simulink model "D_20231120_Modell_Inbetriebnahme_BreakOutBox_Jetson"  (R2022b)
settings: Solver=ode1  StartTime=0.0  StopTime=inf  FixedStep=Ts  RelTol=1e-3
PreLoadFcn:
  | pulsePeriod = 0.05;
  | 
  | Ts = 0.001;
  | 
  | FPGA_Frequency = 75000000;
  | 
  | ts_IO691 = 5e-3;
PostLoadFcn:
  | ewolfSetUp
InitFcn:
  | pulsePeriod = 0.05;
  | 
  | Ts = 0.001;
  | 
  | FPGA_Frequency = 75000000;
  | 
  | ts_IO691 = 5e-3;
StopFcn:
  | Simulink.sdi.clearPreferences;
  | if isfile(['sdi_view_',bdroot,'.mldatx'])
  | Simulink.sdi.view;
  | pause(3);
  | Simulink.sdi.loadView(['sdi_view_',bdroot,]);
  | end
model workspace (MAT data in the model file):
  MaxDreh = 1
values from neighbouring files (symbols this model uses):
  max_ac = 2    [ewolfSetUp.m]
  min_ac = -3    [ewolfSetUp.m]
  PredictionHorizon = 30    [ewolfSetUp.m]
undefined symbols (not defined in the file or in its folder): canChannel, DiscIntNeverNeededParam, Ended, HS, IO291, IO397, max_steer_car, min_steer_car, sigbuilder_block, Single
libraries: lllalib x255, canmsglib x146, simulink x42, speedgoatlib_IO191 x5, speedgoatlib_IO291 x5, slrealtimeiplib x3, speedgoatlib_IO691 x3, slrealtimeutilitieslib x2, spsEdgeDetectorLib x1, simulink_extras x1, speedgoatlib_fpga_dio x1, speedgoatlib_fpga_quadrature x1
(part 7 of 8)

== system D_20231120_Modell_Inbetriebnahme_BreakOutBox_Jetson/Lenkung Steuerung/Beobachter und Begrenzer/Lenkwingelgeschwindigkeitsbegrenzer ==
  "Drehmomvor. norm. " : Inport
  LenkDrehmomentMaxNomiert : Inport  Port=2
  Constant : Constant  Value=0
  Saturation : Saturate  UpperLimit=1  LowerLimit=0
  Saturation Dynamic : simulink/Discontinuities/Saturation Dynamic  OutMin=[]  OutMax=[]  OutDataTypeStr=Inherit: Same as second input  OutDataType=fixdt(1, 16)  OutScaling=2^-10  DoSatur=off
  Saturation1 : Saturate  UpperLimit=1  LowerLimit=0
  Terminator : Terminator
  Drehmoment norm. begr. : Outport
  wires:
  Saturation1/1 -> Drehmoment norm. begr./1
  "Drehmomvor. norm. "/1 -> Saturation Dynamic/2, Saturation1/1
  Constant/1 -> Saturation Dynamic/3
  LenkDrehmomentMaxNomiert/1 -> Saturation/1
  Saturation/1 -> Saturation Dynamic/1
  Saturation Dynamic/1 -> Terminator/1  "Drehmoment norm. begr. Test"

== system D_20231120_Modell_Inbetriebnahme_BreakOutBox_Jetson/Lenkung Steuerung/Beobachter und Begrenzer/Lenkwinkelbegrenzer ==
  Lenkwinkel nomiert : Inport
  Drehmomvor. norm. : Inport  Port=2
  "Maximaler Lenkwinkel normiert und Geschwindigkeitsabhängig " : Inport  Port=3
  Constant : Constant
  Constant1 : Constant  Value=0.5
  IC1 : InitialCondition  Value=0.5
  Lamp : LampBlock  LabelPosition=Hide
  Lamp1 : LampBlock  LabelPosition=Hide
  Lamp2 : LampBlock  LabelPosition=Hide
  RT : RateTransition  OutPortSampleTime=0.001
  Relational Operator : RelationalOperator  OutDataTypeStr=boolean  RndMeth=Simplest  InputSameDT=off
  Relational Operator1 : RelationalOperator  Operator=<=  OutDataTypeStr=boolean  RndMeth=Simplest  InputSameDT=off
  Split pos. and neg. Drehmoment : Subsystem
  Sum : Sum  Inputs=|+-
  Switch : Switch  Criteria=u2 > Threshold  SaturateOnIntegerOverflow=off  InputSameDT=off
  Switch1 : Switch  Criteria=u2 > Threshold  SaturateOnIntegerOverflow=off  InputSameDT=off
  Switch2 : Switch  Criteria=u2 > Threshold  SaturateOnIntegerOverflow=off  InputSameDT=off
  "Drehmomvor. norm. " : Outport
  wires:
  Drehmomvor. norm./1 -> Split pos. and neg. Drehmoment/1(Drehmomvor. norm.)
  Switch/1 -> Switch2/3
  Switch1/1 -> Switch2/1
  Split pos. and neg. Drehmoment/2(bool Welle) -> Switch2/2
  Split pos. and neg. Drehmoment/3(neg. Welle) -> Switch/1
  Relational Operator/1 -> Switch/2
  Relational Operator1/1 -> RT/1
  Lenkwinkel nomiert/1 -> Relational Operator/1, Relational Operator1/1
  "Maximaler Lenkwinkel normiert und Geschwindigkeitsabhängig "/1 -> Sum/2, Relational Operator1/2
  Constant1/1 -> Switch1/3, Switch/3
  RT/1 -> Switch1/2
  Split pos. and neg. Drehmoment/1(pos. Welle) -> Switch1/1
  Sum/1 -> Relational Operator/2
  Constant/1 -> Sum/1
  IC1/1 -> "Drehmomvor. norm. "/1
  Switch2/1 -> IC1/1

== system D_20231120_Modell_Inbetriebnahme_BreakOutBox_Jetson/Lenkung Steuerung/Beobachter und Begrenzer/Subsystem1 ==
  Geschwindigkeit : Inport
  Lenkwinkel : Inport  Port=2
  Constant : Constant  Value=10
  Derivative : Derivative
  MATLAB Function : MATLAB Function  TreatAsAtomicUnit=on
  MATLAB Function1 : MATLAB Function  TreatAsAtomicUnit=on
  Product : Product
  lenkradwinkelMaxNomiert : Outport
  LenkDrehmomentMaxNomiert : Outport  Port=2
  wires:
  MATLAB Function1/1(LenkDrehmomentMaxNomiert) -> LenkDrehmomentMaxNomiert/1  "LenkDrehmomentMaxNomiert"
  MATLAB Function/1(lenkradwinkelMaxNomiert) -> lenkradwinkelMaxNomiert/1  "lenkradwinkelMaxNomiert"
  Lenkwinkel/1 -> MATLAB Function/1(Lenkwinkel), Derivative/1
  Derivative/1 -> MATLAB Function1/1(Lenkwinkelgeschwindigkeit)  "LenkradwinkelGeschwindigkeit"
  Geschwindigkeit/1 -> Product/1
  Product/1 -> MATLAB Function/2(Fahrzeuggeschwindigkeit), MATLAB Function1/2(Fahrzeuggeschwindigkeit)
  Constant/1 -> Product/2

== system D_20231120_Modell_Inbetriebnahme_BreakOutBox_Jetson/Lenkung Steuerung/Lenkmomentsimulationssignalgeber/Signal Builder ==
  Demux : Demux  Tag=STV Demux  Outputs=5
      settings: DisplayOption=none
  FromWs : FromWorkspace  Tag=STV FromWs  VariableName=tuvar
      SigBuilderData=|
      | common.afterFinalStr = 'Extrapolate'
      | common.sampleTime = 0
      | dataSet.timeRange = [0 100]
      | dataSet.name = 'Group 1'
      | sbobj.Groups.Name = 'Group 1'
      | sbobj.Groups.Signals(1).Name = 'Signal 1'
      | sbobj.Groups.Signals(1).XData = [0 5 5 10 10 15 15 20 20 25 25 30 30 35 35 40 40 45 45 50 50 55 55 60 60 65 65 70 70 75 75 80 80 85 85 90 90 95 95 100]
      | sbobj.Groups.Signals(1).YData = [0 0 0.5 0.5 0 0 -0.5 -0.5 0 0 1 1 0 0 -1 -1 0 0 1.5 1.5 0 0 -1.5 -1.5 0 0 2 2 0 0 -2 -2 -0.05 -0.05 0.25 0.25 0 0 -0.25 -0.25]
      | sbobj.Groups.Signals(2).Name = 'Signal 2'
      | sbobj.Groups.Signals(2).XData = [0 10 10 30 30 100]
      | sbobj.Groups.Signals(2).YData = [0.5 0.5 0.3 0.3 0.7 0.7]
      | sbobj.Groups.Signals(3).Name = 'Signal 3'
      | sbobj.Groups.Signals(3).XData = [0 20 40 40 60 100]
      | sbobj.Groups.Signals(3).YData = [0.5 0.5 1 0.5 0 0.5]
      | sbobj.Groups.Signals(4).Name = 'Signal 4'
      | sbobj.Groups.Signals(4).XData = [0 10 10 100]
      | sbobj.Groups.Signals(4).YData = [0 0 0.5 0.5]
      | sbobj.Groups.Signals(5).Name = 'Signal 5'
      | sbobj.Groups.Signals(5).XData = [0 20 100]
      | sbobj.Groups.Signals(5).YData = [-4 -4 4]
      | sbobj.Groups.TimeRange = [0 100]
  Signal 1 : Outport  Tag=STV Outport
  Signal 2 : Outport  Tag=STV Outport  Port=2
  Signal 3 : Outport  Tag=STV Outport  Port=3
  Signal 4 : Outport  Tag=STV Outport  Port=4
  Signal 5 : Outport  Tag=STV Outport  Port=5
  wires:
  Demux/1 -> Signal 1/1
  FromWs/1 -> Demux/1
  Demux/2 -> Signal 2/1
  Demux/3 -> Signal 3/1
  Demux/4 -> Signal 4/1
  Demux/5 -> Signal 5/1

== system D_20231120_Modell_Inbetriebnahme_BreakOutBox_Jetson/Nvidia_Jetson/LaneFollowingAndControl/Estimate Lane Center1 ==
  note: Estimate Lane Center
  Lane Detections : Inport
  Longitudinal Velocity : Inport  Port=2
  Center from Left and Right1 : Subsystem  TreatAsAtomicUnit=on
  Center from Left1 : Subsystem  TreatAsAtomicUnit=on
  Center from None1 : Subsystem  TreatAsAtomicUnit=on
  Center from Right1 : Subsystem  TreatAsAtomicUnit=on
  Delay1 : Delay  DelayLength=1
  Lane Detections5 : InportShadow
  Lane Detections6 : InportShadow
  Lane Detections7 : InportShadow
  MATLAB Function1 : MATLAB Function  TreatAsAtomicUnit=on
  Merge1 : Merge  Inputs=4
  Preview Curvature : Subsystem  VariantControl=v2
      settings: RTWFileNameOpts=Use function name
  Previewed Curvature : Outport  VectorParamsAs1DForOutWhenUnconnected=off
  Lateral Offset : Outport  Port=2  VectorParamsAs1DForOutWhenUnconnected=off
  Heading Angle : Outport  Port=3  VectorParamsAs1DForOutWhenUnconnected=off
  wires:
  Preview Curvature/1(Previewed Curvature) -> Previewed Curvature/1
  Merge1/1 -> Preview Curvature/1(Lane Center), Delay1/1
  Center from Left1/1(Center) -> Merge1/2
  Lane Detections5/1 -> Center from Left and Right1/1(Lanes)
  Center from Left and Right1/1(Center) -> Merge1/1
  Lane Detections6/1 -> Center from Left1/1(Lanes)
  Delay1/1 -> Center from None1/1(In1)
  Lane Detections/1 -> MATLAB Function1/1(lanes)
  Lane Detections7/1 -> Center from Right1/1(Lanes)
  Center from None1/1(Out1) -> Merge1/4
  Center from Right1/1(Center) -> Merge1/3
  Longitudinal Velocity/1 -> Preview Curvature/2(Longitudinal Velocity)
  Preview Curvature/3(Relative Yaw Angle) -> Heading Angle/1  "relative_yaw_angle"
  Preview Curvature/2(Lateral Deviation) -> Lateral Offset/1  "lateral_deviation"
  MATLAB Function1/1(fcnLeftAndRight()) -> Center from Left and Right1/Trigger
  MATLAB Function1/2(fcnLeftOnly()) -> Center from Left1/Trigger
  MATLAB Function1/3(fcnRightOnly()) -> Center from Right1/Trigger
  MATLAB Function1/4(fcnNone()) -> Center from None1/Trigger

== system D_20231120_Modell_Inbetriebnahme_BreakOutBox_Jetson/Nvidia_Jetson/LaneFollowingAndControl/MPC Controller ==
  Set velocity : Inport
  Longitudinal velocity : Inport  Port=2
  Curvature : Inport  Port=3
  Lateral deviation : Inport  Port=4
  Relative yaw angle : Inport  Port=5
  Initial Velocity : Constant  Value=0.1
  Path Following Control System : mpcadaslib/Path Following Control System  VariantControl=Variant2  ModelType=Use vehicle parameters  VehicleMass=m  VehicleYawInertia=Iz  LengthToFront=lf  LengthToRear=lr  FrontTireStiffness=Cf  RearTireStiffness=Cr  AccelTimeConstant=tau  EgoModelMatrixA=[-2,zeros(1,3);1,zeros(1,3);zeros(1,2),-4.4021,-12.4603;zeros(1,2),1.3913,-5.1868]  EgoModelMatrixB=[2,zeros(1,3);zeros(1,2),24.1270,15.8609]'  EgoModelMatrixC=[zeros(3,1),eye(3)]  InitialLongVel=v0_ego  TransportLag=0.1  spaceCtrl=off  DefaultSpacing=default_spacing  MinSteering=min_steer  umin_ext=off  MaxSteering=max_steer  umax_ext=off  MinAcceleration=min_ac  amin_ext=off  MaxAcceleration=max_ac  amax_ext=off  Ts=0.1  PredictionHorizon=PredictionHorizon  ControlHorizon=2  LongWeight=0.1  LateralWeight=1  AccelRateWeight=0.1  SteerRateWeight=0.1  suboptimal=off  maxiter=10  datatypeopt=double  optmode=off  trackmode=off
  Switch : Switch  Criteria=u2 > Threshold  Threshold=0.1  SaturateOnIntegerOverflow=off  InputSameDT=off
  Steering Angle : Outport  VectorParamsAs1DForOutWhenUnconnected=off
  Acceleration : Outport  Port=2  VectorParamsAs1DForOutWhenUnconnected=off
  wires:
  Lateral deviation/1 -> Path Following Control System/4
  Curvature/1 -> Path Following Control System/3
  Set velocity/1 -> Path Following Control System/1
  Path Following Control System/2 -> Steering Angle/1
  Path Following Control System/1 -> Acceleration/1
  Relative yaw angle/1 -> Path Following Control System/5
  Initial Velocity/1 -> Switch/3
  Longitudinal velocity/1 -> Switch/2, Switch/1  "Longitudinal_Velocity"
  Switch/1 -> Path Following Control System/2

== system D_20231120_Modell_Inbetriebnahme_BreakOutBox_Jetson/Freigabe/Freigabe/Detektion Fahrpedal/Moving Average ==
  In : Inport
  Divide : Product  Inputs=*/
  Sum of Elements : Sum  Inputs=+
  Tapped Delay : simulink/Discrete/Tapped Delay  vinit=0.0  samptime=-1  NumDelays=4  DelayOrder=Oldest  includeCurrent=off
  Vector Concatenate : Concatenate
  Width : Width
  Out : Outport
  wires:
  In/1 -> Vector Concatenate/1, Tapped Delay/1
  Sum of Elements/1 -> Divide/1
  Width/1 -> Divide/2
  Vector Concatenate/1 -> Sum of Elements/1, Width/1
  Divide/1 -> Out/1
  Tapped Delay/1 -> Vector Concatenate/2

== system D_20231120_Modell_Inbetriebnahme_BreakOutBox_Jetson/Freigabe/Freigabe/Detektion Fahrpedal/Moving Average1 ==
  In : Inport
  Divide : Product  Inputs=*/
  Sum of Elements : Sum  Inputs=+
  Tapped Delay : simulink/Discrete/Tapped Delay  vinit=0.0  samptime=-1  NumDelays=4  DelayOrder=Oldest  includeCurrent=off
  Vector Concatenate : Concatenate
  Width : Width
  Out : Outport
  wires:
  In/1 -> Vector Concatenate/1, Tapped Delay/1
  Sum of Elements/1 -> Divide/1
  Width/1 -> Divide/2
  Vector Concatenate/1 -> Sum of Elements/1, Width/1
  Divide/1 -> Out/1
  Tapped Delay/1 -> Vector Concatenate/2

== system D_20231120_Modell_Inbetriebnahme_BreakOutBox_Jetson/IO691/CAN Read Loop - Port 3/Enabled Subsystem/extract radar data from CAN msg stream ==
  msg : Inport
  CAN Log : canlib/CAN Log  Commented=on  BlockHandle=781.0001  FullPathFileName=loGG.mat  FileName=loGG.mat  VariableName=saveMSG  MaxNumMessages=1000  LogFrom=CAN Bus  DeviceMenu=Select a device  Device=Vector CANcaseXL 1 (Channel 1)  ObjConstructor=canChannel('Vector', 'CANcaseXL 1', 1)  SampleTime=inf
  Mux : Mux  Inputs=6
  Subsystem1 : Subsystem
  Subsystem100 : Subsystem
  extract point from CAN msg : Subsystem
  save 55 : Subsystem
  enable outP : Outport
  data : Outport  Port=2  OutDataTypeStr=double
  Radar_Punkt : Outport  Port=3
  Radar_Mode : Outport  Port=4
  wires:
  extract point from CAN msg/6(numobj) -> Mux/3
  extract point from CAN msg/4(cycle) -> Mux/2
  extract point from CAN msg/3(data) -> Radar_Punkt/1, Subsystem100/2(data)
  extract point from CAN msg/2(timestamp) -> Mux/1
  msg/1 -> extract point from CAN msg/1(msg)
  extract point from CAN msg/1(enable) -> Subsystem100/1(reset), Subsystem1/1(reset), save 55/1(reset), enable outP/1
  extract point from CAN msg/5(mode) -> Subsystem100/3(saveBool), Subsystem1/3(saveBool), save 55/3(saveBool), Radar_Mode/1
  Mux/1 -> data/1
  Subsystem100/1(Out1) -> Mux/4
  save 55/1(Out1) -> Mux/6
  Subsystem1/1(Out1) -> Mux/5
  Subsystem1/2(nextSave) -> save 55/2(data)
  Subsystem100/2(nextSave) -> Subsystem1/2(data)

== system D_20231120_Modell_Inbetriebnahme_BreakOutBox_Jetson/Lenkung Steuerung/Beobachter und Begrenzer/Lenkwinkelbegrenzer/Split pos. and neg. Drehmoment ==
  Drehmomvor. norm. : Inport
  Constant : Constant  Value=0.5
  Enabled Subsystem : Subsystem  TreatAsAtomicUnit=on
  Enabled Subsystem1 : Subsystem  TreatAsAtomicUnit=on
  Logical Operator : Logic  Operator=NOT  AllPortsSameDT=off  OutDataTypeStr=boolean
  Relational Operator : RelationalOperator  Operator=>  OutDataTypeStr=boolean  RndMeth=Simplest  InputSameDT=off
  pos. Welle : Outport
  bool Welle : Outport  Port=2
  neg. Welle : Outport  Port=3
  wires:
  Relational Operator/1 -> bool Welle/1, Logical Operator/1, Enabled Subsystem1/Enable
  Drehmomvor. norm./1 -> Enabled Subsystem/1(Drehmomentsvorgabe normiert), Relational Operator/1, Enabled Subsystem1/1(Drehmomentsvorgabe normiert)
  Constant/1 -> Relational Operator/2
  Logical Operator/1 -> Enabled Subsystem/Enable
  Enabled Subsystem1/1(Out1) -> pos. Welle/1
  Enabled Subsystem/1(Out1) -> neg. Welle/1

== system D_20231120_Modell_Inbetriebnahme_BreakOutBox_Jetson/Nvidia_Jetson/LaneFollowingAndControl/Estimate Lane Center1/Center from Left and Right1 ==
  note: Center from Left and Right
  In Bus Element : Inport  PortName=Lanes  Element=Left.Curvature
  In Bus Element2 : Inport  PortName=Lanes  Element=Left.CurvatureDerivative
  In Bus Element4 : Inport  PortName=Lanes  Element=Left.HeadingAngle
  In Bus Element6 : Inport  PortName=Lanes  Element=Left.LateralOffset
  In Bus Element1 : Inport  PortName=Lanes  Element=Right.Curvature
  In Bus Element3 : Inport  PortName=Lanes  Element=Right.CurvatureDerivative
  In Bus Element5 : Inport  PortName=Lanes  Element=Right.HeadingAngle
  In Bus Element7 : Inport  PortName=Lanes  Element=Right.LateralOffset
  function : TriggerPort  TriggerType=function-call  VariantControl=Variant
  Add{,1..3} (4 alike) : Sum
  Bus Creator : BusCreator  Inputs=4
  Gain{,1..3} (4 alike) : Gain  Gain=0.5
  Center : Outport  VectorParamsAs1DForOutWhenUnconnected=off
  wires:
  In Bus Element6/1 -> Add3/1
  In Bus Element7/1 -> Add3/2
  In Bus Element5/1 -> Add2/2
  In Bus Element4/1 -> Add2/1
  In Bus Element3/1 -> Add1/2
  In Bus Element2/1 -> Add1/1
  In Bus Element1/1 -> Add/2
  In Bus Element/1 -> Add/1
  Bus Creator/1 -> Center/1
  Gain3/1 -> Bus Creator/4  "LateralOffset"
  Add3/1 -> Gain3/1
  Gain2/1 -> Bus Creator/3  "HeadingAngle"
  Add2/1 -> Gain2/1
  Gain1/1 -> Bus Creator/2  "CurvatureDerivative"
  Add1/1 -> Gain1/1
  Gain/1 -> Bus Creator/1  "Curvature"
  Add/1 -> Gain/1

== system D_20231120_Modell_Inbetriebnahme_BreakOutBox_Jetson/Nvidia_Jetson/LaneFollowingAndControl/Estimate Lane Center1/Center from Left1 ==
  note: Curvature Derivative
      | = D[ 1 / ( 1 / (left curvature) – guard)]
      | = left curvature derivative / (1 – (left curvature) * guard)^2.
  note: Center from Left
  note: Curvature
      | = 1 / ( 1 / (left curvature) – guard)
      | = left curvature / (1 – (left curvature) * guard).
  In Bus Element : Inport  PortName=Lanes  Element=Left.Curvature
  In Bus Element2 : Inport  PortName=Lanes  Element=Left.CurvatureDerivative
  In Bus Element4 : Inport  PortName=Lanes  Element=Left.HeadingAngle
  In Bus Element6 : Inport  PortName=Lanes  Element=Left.LateralOffset
  function : TriggerPort  TriggerType=function-call  VariantControl=Variant
  Bus Creator : BusCreator  Inputs=4
  Constant : Constant  OutDataTypeStr=Inherit: Inherit via back propagation
  Divide : Product  Inputs=*/
  Divide1 : Product  Inputs=*/
  Half Lane Width Estimate : Constant  Value=1.8  OutDataTypeStr=Inherit: Inherit via back propagation
  Half Lane Width Estimate1 : Constant  Value=1.8  OutDataTypeStr=Inherit: Inherit via back propagation
  Product : Product
  Product1 : Product
  Subtract : Sum  Inputs=+-
  Subtract1 : Sum  Inputs=+-
  Center : Outport  VectorParamsAs1DForOutWhenUnconnected=off
  wires:
  Product/1 -> Subtract/2
  Half Lane Width Estimate1/1 -> Subtract1/2
  In Bus Element6/1 -> Subtract1/1  "LateralOffset"
  Product1/1 -> Divide1/2
  In Bus Element2/1 -> Divide1/1  "CurvatureDerivative"
  Constant/1 -> Subtract/1
  Half Lane Width Estimate/1 -> Product/2
  Subtract/1 -> Divide/2, Product1/1, Product1/2
  In Bus Element/1 -> Divide/1, Product/1  "Curvature"
  Subtract1/1 -> Bus Creator/4  "LateralOffset"
  In Bus Element4/1 -> Bus Creator/3  "HeadingAngle"
  Divide/1 -> Bus Creator/1  "Curvature"
  Divide1/1 -> Bus Creator/2  "CurvatureDerivative"
  Bus Creator/1 -> Center/1

== system D_20231120_Modell_Inbetriebnahme_BreakOutBox_Jetson/Nvidia_Jetson/LaneFollowingAndControl/Estimate Lane Center1/Center from None1 ==
  In1 : Inport
  function : TriggerPort  TriggerType=function-call  VariantControl=Variant
  Out1 : Outport  VectorParamsAs1DForOutWhenUnconnected=off
  wires:
  In1/1 -> Out1/1

== system D_20231120_Modell_Inbetriebnahme_BreakOutBox_Jetson/Nvidia_Jetson/LaneFollowingAndControl/Estimate Lane Center1/Center from Right1 ==
  note: Curvature Derivative
      | = D[ 1 / ( 1 / (right curvature) + guard)]
      | = right curvature derivative / (1 + (right curvature) * guard)^2
  note: Curvature
      | = 1 / ( 1 / (right curvature) + guard)
      | = right curvature / (1 + (right curvature) * guard)
  note: Center from Right
  In Bus Element : Inport  PortName=Lanes  Element=Right.Curvature
  In Bus Element2 : Inport  PortName=Lanes  Element=Right.CurvatureDerivative
  In Bus Element4 : Inport  PortName=Lanes  Element=Right.HeadingAngle
  In Bus Element6 : Inport  PortName=Lanes  Element=Right.LateralOffset
  function : TriggerPort  TriggerType=function-call  VariantControl=Variant
  Bus Creator : BusCreator  Inputs=4
  Constant : Constant  OutDataTypeStr=Inherit: Inherit via back propagation
  Divide : Product  Inputs=*/
  Divide1 : Product  Inputs=*/
  Half Lane Width Estimate : Constant  Value=1.8  OutDataTypeStr=Inherit: Inherit via back propagation
  Half Lane Width Estimate1 : Constant  Value=1.8  OutDataTypeStr=Inherit: Inherit via back propagation
  Product : Product
  Product1 : Product
  Subtract : Sum
  Subtract1 : Sum
  Center : Outport  VectorParamsAs1DForOutWhenUnconnected=off
  wires:
  Half Lane Width Estimate/1 -> Product/2
  Product/1 -> Subtract/2
  Constant/1 -> Subtract/1
  Subtract/1 -> Divide/2, Product1/1, Product1/2
  In Bus Element/1 -> Divide/1, Product/1  "Curvature"
  Bus Creator/1 -> Center/1
  Subtract1/1 -> Bus Creator/4  "LateralOffset"
  Divide/1 -> Bus Creator/1  "Curvature"
  In Bus Element6/1 -> Subtract1/1  "LateralOffset"
  Half Lane Width Estimate1/1 -> Subtract1/2
  In Bus Element4/1 -> Bus Creator/3  "HeadingAngle"
  Product1/1 -> Divide1/2
  Divide1/1 -> Bus Creator/2  "CurvatureDerivative"
  In Bus Element2/1 -> Divide1/1  "CurvatureDerivative"

== system D_20231120_Modell_Inbetriebnahme_BreakOutBox_Jetson/Nvidia_Jetson/LaneFollowingAndControl/Estimate Lane Center1/Preview Curvature ==
  Lane Center : Inport
  Longitudinal Velocity : Inport  Port=2
  Bus Selector : BusSelector  OutputSignals=Curvature,CurvatureDerivative,HeadingAngle,LateralOffset
  Data Type Conversion{,1..3} (4 alike) : DataTypeConversion  SaturateOnIntegerOverflow=off  RndMeth=Floor
  Gain : Gain  Gain=[0:0.1:PredictionHorizon*0.1]'
      settings: AttributesFormatString=|
      | ----------------------------------------
      | Gain = %<Gain>
  ISO 8855 to SAE J670E : Subsystem
  Product : Product
  Saturation : Saturate
      settings: AttributesFormatString=|
      | -------------------------------
      | UpperLimit = %<UpperLimit>
      | LowerLimit = %<LowerLimit>
  Saturation1 : Saturate  UpperLimit=0.6  LowerLimit=-0.6
      settings: AttributesFormatString=|
      | -------------------------------
      | UpperLimit = %<UpperLimit>
      | LowerLimit = %<LowerLimit>
  Saturation2 : Saturate  UpperLimit=0.15  LowerLimit=-0.15
      settings: AttributesFormatString=|
      | -------------------------------
      | UpperLimit = %<UpperLimit>
      | LowerLimit = %<LowerLimit>
  Saturation3 : Saturate  UpperLimit=0.06  LowerLimit=-0.06
      settings: AttributesFormatString=|
      | -------------------------------
      | UpperLimit = %<UpperLimit>
      | LowerLimit = %<LowerLimit>
  Sum : Sum
  Unary Minus : UnaryMinus
  Unary Minus1 : UnaryMinus
  Previewed Curvature : Outport  VectorParamsAs1DForOutWhenUnconnected=off
  Lateral Deviation : Outport  Port=2  VectorParamsAs1DForOutWhenUnconnected=off
  Relative Yaw Angle : Outport  Port=3  VectorParamsAs1DForOutWhenUnconnected=off
  wires:
  Lane Center/1 -> ISO 8855 to SAE J670E/1(ISO)
  ISO 8855 to SAE J670E/1(SAE) -> Bus Selector/1
  Bus Selector/3 -> Data Type Conversion/1  "<HeadingAngle>"
  Bus Selector/4 -> Data Type Conversion1/1  "<LateralOffset>"
  Unary Minus1/1 -> Saturation/1
  Bus Selector/1 -> Data Type Conversion3/1  "<Curvature>"
  Bus Selector/2 -> Data Type Conversion2/1  "<CurvatureDerivative>"
  Longitudinal Velocity/1 -> Product/2
  Unary Minus/1 -> Saturation1/1
  Saturation/1 -> Lateral Deviation/1
  Saturation1/1 -> Relative Yaw Angle/1
  Saturation3/1 -> Product/1
  Product/1 -> Gain/1
  Sum/1 -> Previewed Curvature/1
  Gain/1 -> Sum/2
  Saturation2/1 -> Sum/1
  Data Type Conversion/1 -> Unary Minus/1
  Data Type Conversion1/1 -> Unary Minus1/1
  Data Type Conversion2/1 -> Saturation3/1
  Data Type Conversion3/1 -> Saturation2/1

== system D_20231120_Modell_Inbetriebnahme_BreakOutBox_Jetson/IO691/CAN Read Loop - Port 3/Enabled Subsystem/extract radar data from CAN msg stream/Subsystem1 ==
  reset : Inport
  data : Inport  Port=2
  saveBool : Inport  Port=3
  Mux : Mux  Inputs=10
  Subsystem : Subsystem
  Subsystem1 : Subsystem
  Subsystem2 : Subsystem
  Subsystem3 : Subsystem
  Subsystem4 : Subsystem
  Subsystem5 : Subsystem
  Subsystem6 : Subsystem
  Subsystem7 : Subsystem
  Subsystem8 : Subsystem
  Subsystem9 : Subsystem
  Out1 : Outport
  nextSave : Outport  Port=2
  wires:
  Subsystem4/1(out) -> Mux/5
  Mux/1 -> Out1/1
  Subsystem1/1(out) -> Mux/2
  Subsystem7/2(nextSave) -> Subsystem8/2(data)
  Subsystem8/2(nextSave) -> Subsystem9/2(data)
  Subsystem2/1(out) -> Mux/3
  Subsystem6/1(out) -> Mux/7
  data/1 -> Subsystem/2(data)
  Subsystem9/2(nextSave) -> nextSave/1
  Subsystem6/2(nextSave) -> Subsystem7/2(data)
  Subsystem5/2(nextSave) -> Subsystem6/2(data)
  Subsystem/1(out) -> Mux/1
  Subsystem9/1(out) -> Mux/10
  Subsystem3/1(out) -> Mux/4
  Subsystem5/1(out) -> Mux/6
  Subsystem2/2(nextSave) -> Subsystem3/2(data)
  Subsystem7/1(out) -> Mux/8
  Subsystem3/2(nextSave) -> Subsystem4/2(data)
  Subsystem8/1(out) -> Mux/9
  Subsystem1/2(nextSave) -> Subsystem2/2(data)
  Subsystem/2(nextSave) -> Subsystem1/2(data)
  Subsystem4/2(nextSave) -> Subsystem5/2(data)
  reset/1 -> Subsystem9/1(reset), Subsystem8/1(reset), Subsystem7/1(reset), Subsystem6/1(reset), Subsystem5/1(reset), Subsystem4/1(reset), Subsystem3/1(reset), Subsystem2/1(reset), Subsystem1/1(reset), Subsystem/1(reset)
  saveBool/1 -> Subsystem/3(saveBool), Subsystem1/3(saveBool), Subsystem3/3(saveBool), Subsystem9/3(saveBool), Subsystem8/3(saveBool), Subsystem7/3(saveBool), Subsystem6/3(saveBool), Subsystem5/3(saveBool), Subsystem4/3(saveBool), Subsystem2/3(saveBool)

== system D_20231120_Modell_Inbetriebnahme_BreakOutBox_Jetson/IO691/CAN Read Loop - Port 3/Enabled Subsystem/extract radar data from CAN msg stream/Subsystem100 ==
  reset : Inport
  data : Inport  Port=2
  saveBool : Inport  Port=3
  Mux : Mux  Inputs=10
  Subsystem : Subsystem
  Subsystem1 : Subsystem
  Subsystem2 : Subsystem
  Subsystem3 : Subsystem
  Subsystem4 : Subsystem
  Subsystem5 : Subsystem
  Subsystem6 : Subsystem
  Subsystem7 : Subsystem
  Subsystem8 : Subsystem
  Subsystem9 : Subsystem
  Out1 : Outport
  nextSave : Outport  Port=2
  wires:
  Subsystem4/1(out) -> Mux/5
  Mux/1 -> Out1/1
  Subsystem1/1(out) -> Mux/2
  Subsystem7/2(nextSave) -> Subsystem8/2(data)
  Subsystem8/2(nextSave) -> Subsystem9/2(data)
  Subsystem2/1(out) -> Mux/3
  Subsystem6/1(out) -> Mux/7
  data/1 -> Subsystem/2(data)
  Subsystem9/2(nextSave) -> nextSave/1
  Subsystem6/2(nextSave) -> Subsystem7/2(data)
  Subsystem5/2(nextSave) -> Subsystem6/2(data)
  Subsystem/1(out) -> Mux/1
  Subsystem9/1(out) -> Mux/10
  Subsystem3/1(out) -> Mux/4
  Subsystem5/1(out) -> Mux/6
  Subsystem2/2(nextSave) -> Subsystem3/2(data)
  Subsystem7/1(out) -> Mux/8
  Subsystem3/2(nextSave) -> Subsystem4/2(data)
  Subsystem8/1(out) -> Mux/9
  Subsystem1/2(nextSave) -> Subsystem2/2(data)
  Subsystem/2(nextSave) -> Subsystem1/2(data)
  Subsystem4/2(nextSave) -> Subsystem5/2(data)
  reset/1 -> Subsystem9/1(reset), Subsystem8/1(reset), Subsystem7/1(reset), Subsystem6/1(reset), Subsystem5/1(reset), Subsystem4/1(reset), Subsystem3/1(reset), Subsystem2/1(reset), Subsystem1/1(reset), Subsystem/1(reset)
  saveBool/1 -> Subsystem/3(saveBool), Subsystem1/3(saveBool), Subsystem3/3(saveBool), Subsystem9/3(saveBool), Subsystem8/3(saveBool), Subsystem7/3(saveBool), Subsystem6/3(saveBool), Subsystem5/3(saveBool), Subsystem4/3(saveBool), Subsystem2/3(saveBool)

== system D_20231120_Modell_Inbetriebnahme_BreakOutBox_Jetson/IO691/CAN Read Loop - Port 3/Enabled Subsystem/extract radar data from CAN msg stream/extract point from CAN msg ==
  msg : Inport
  Constant : Constant
  Constant1 : Constant  Value=0
  Terminator{,1..3} (4 alike) : Terminator
  extract radar_CAN_data (each cycle) : Subsystem  TreatAsAtomicUnit=on
  extract_header_info : canmsglib/CAN Unpack  MsgList=(none)  MsgName=CAN Msg  MsgIDType=Standard (11-bit identifier)  MsgIdentifier=1024  MsgLength=8  SignalInfo={ 'dur', '0', '11', 'LE', 'unsigned', 'Standard', '0', '1', '0', '-Inf', 'Inf'; 'Signal2', '12', '3', 'LE', 'unsigned', 'Standard', '0', '1', '0', '-Inf', 'Inf'; 'cycl_count', '15', '31', 'LE', 'unsigned', 'Standard', '0', '1', '0', '-Inf', 'Inf'; 'numObj', '47', '7', 'LE', 'unsigned', 'Standard', '0', '1', '0', '-Inf', 'Inf'; 'Signal5', '55', '8', 'LE', 'unsigned', 'Standard', '0', '1', '0', '-Inf', 'Inf' }  IDPort=off  TimestampPort=on  ErrorPort=off  RemotePort=off  LengthPort=off  StatusPort=on  ApplyMinMax=off
  if_header_msg : MATLAB Function  TreatAsAtomicUnit=on
  switch between header = enable and not : MultiPortSwitch  DataPortOrder=Specify indices  DataPortIndices={1,0}  OutDataTypeStr=uint32  SaturateOnIntegerOverflow=off  InputSameDT=off
  enable : Outport
  timestamp : Outport  Port=2
  data : Outport  Port=3
  cycle : Outport  Port=4
  mode : Outport  Port=5
  numobj : Outport  Port=6
  wires:
  switch between header = enable and not/1 -> enable/1
  extract radar_CAN_data (each cycle)/3(mode) -> mode/1
  extract_header_info/6 -> timestamp/1
  if_header_msg/1(isHeader) -> switch between header = enable and not/1
  extract_header_info/4 -> numobj/1, if_header_msg/3(numObj)
  Constant1/1 -> switch between header = enable and not/3
  Constant/1 -> switch between header = enable and not/2
  extract radar_CAN_data (each cycle)/2(data) -> data/1
  extract_header_info/3 -> if_header_msg/2(cycl), extract radar_CAN_data (each cycle)/1(cycle_in)
  extract radar_CAN_data (each cycle)/1(cycle) -> cycle/1
  msg/1 -> extract_header_info/1, if_header_msg/1(msg), extract radar_CAN_data (each cycle)/2(msg)
  extract_header_info/1 -> Terminator/1
  extract_header_info/2 -> Terminator1/1
  extract_header_info/5 -> Terminator2/1
  extract_header_info/7 -> Terminator3/1

== system D_20231120_Modell_Inbetriebnahme_BreakOutBox_Jetson/IO691/CAN Read Loop - Port 3/Enabled Subsystem/extract radar data from CAN msg stream/save 55 ==
  reset : Inport
  data : Inport  Port=2
  saveBool : Inport  Port=3
  Mux : Mux  Inputs=6
  Subsystem : Subsystem
  Subsystem1 : Subsystem
  Subsystem2 : Subsystem
  Subsystem3 : Subsystem
  Subsystem4 : Subsystem
  Subsystem5 : Subsystem
  Out1 : Outport
  wires:
  Subsystem4/1(out) -> Mux/5
  Mux/1 -> Out1/1
  Subsystem1/1(out) -> Mux/2
  Subsystem2/1(out) -> Mux/3
  data/1 -> Subsystem/2(data)
  Subsystem/1(out) -> Mux/1
  Subsystem3/1(out) -> Mux/4
  Subsystem5/1(out) -> Mux/6
  Subsystem2/2(nextSave) -> Subsystem3/2(data)
  Subsystem3/2(nextSave) -> Subsystem4/2(data)
  Subsystem1/2(nextSave) -> Subsystem2/2(data)
  Subsystem/2(nextSave) -> Subsystem1/2(data)
  Subsystem4/2(nextSave) -> Subsystem5/2(data)
  reset/1 -> Subsystem5/1(reset), Subsystem4/1(reset), Subsystem3/1(reset), Subsystem2/1(reset), Subsystem1/1(reset), Subsystem/1(reset)
  saveBool/1 -> Subsystem/3(saveBool), Subsystem1/3(saveBool), Subsystem3/3(saveBool), Subsystem5/3(saveBool), Subsystem4/3(saveBool), Subsystem2/3(saveBool)

== system D_20231120_Modell_Inbetriebnahme_BreakOutBox_Jetson/Lenkung Steuerung/Beobachter und Begrenzer/Lenkwinkelbegrenzer/Split pos. and neg. Drehmoment/Enabled Subsystem ==
  Drehmomentsvorgabe normiert : Inport
  Enable : EnablePort
  Out1 : Outport
  wires:
  Drehmomentsvorgabe normiert/1 -> Out1/1

== system D_20231120_Modell_Inbetriebnahme_BreakOutBox_Jetson/Lenkung Steuerung/Beobachter und Begrenzer/Lenkwinkelbegrenzer/Split pos. and neg. Drehmoment/Enabled Subsystem1 ==
  Drehmomentsvorgabe normiert : Inport
  Enable : EnablePort
  Out1 : Outport
  wires:
  Drehmomentsvorgabe normiert/1 -> Out1/1

== system D_20231120_Modell_Inbetriebnahme_BreakOutBox_Jetson/Nvidia_Jetson/LaneFollowingAndControl/Estimate Lane Center1/Preview Curvature/ISO 8855 to SAE J670E ==
  note: ISO 8855 to SAE J670E
  note: positive Y is to the left in ISO 8855
      | positive Y is to the right in SAE J670E
  ISO : Inport
  Bus Creator : BusCreator  Inputs=4
  Bus Selector : BusSelector  OutputSignals=CurvatureDerivative,Curvature,HeadingAngle,LateralOffset
  Signal Specification : SignalSpecification  Unit=1/m^2
  Signal Specification1 : SignalSpecification  Unit=1/m
  Signal Specification2 : SignalSpecification  Unit=rad
  Signal Specification3 : SignalSpecification  Unit=m
  Unary Minus{,1..3} (4 alike) : UnaryMinus
  SAE : Outport  VectorParamsAs1DForOutWhenUnconnected=off
  wires:
  Signal Specification3/1 -> Bus Creator/4  "LateralOffset"
  Signal Specification2/1 -> Bus Creator/3  "HeadingAngle"
  Signal Specification1/1 -> Bus Creator/1  "CurvatureDerivative"
  Unary Minus/1 -> Signal Specification/1
  Unary Minus3/1 -> Signal Specification3/1
  Unary Minus2/1 -> Signal Specification2/1
  Unary Minus1/1 -> Signal Specification1/1
  Signal Specification/1 -> Bus Creator/2  "Curvature"
  Bus Creator/1 -> SAE/1
  Bus Selector/4 -> Unary Minus3/1  "<LateralOffset>"
  Bus Selector/3 -> Unary Minus2/1  "<HeadingAngle>"
  Bus Selector/1 -> Unary Minus1/1  "<CurvatureDerivative>"
  Bus Selector/2 -> Unary Minus/1  "<Curvature>"
  ISO/1 -> Bus Selector/1

== system D_20231120_Modell_Inbetriebnahme_BreakOutBox_Jetson/IO691/CAN Read Loop - Port 3/Enabled Subsystem/extract radar data from CAN msg stream/Subsystem1/Subsystem ==
  reset : Inport
  data : Inport  Port=2
  saveBool : Inport  Port=3
  Mux : Mux  Inputs=10
  saveData{,1..9} (10 alike) : lllalib/saveData  SystemSampleTime=-1  VariantActivationTime=update diagram  Latency=0  AutoFrameSizeCalculation=off
  out : Outport
  nextSave : Outport  Port=2
  wires:
  saveData3/2 -> Mux/4
  saveData8/1 -> saveData9/2
  saveData7/1 -> saveData8/2
  reset/1 -> saveData/1, saveData1/1, saveData2/1, saveData3/1, saveData4/1, saveData5/1, saveData6/1, saveData8/1, saveData9/1, saveData7/1
  saveData3/1 -> saveData4/2
  saveData4/1 -> saveData5/2
  saveData2/2 -> Mux/3
  Mux/1 -> out/1
  saveData6/2 -> Mux/7
  saveData9/1 -> nextSave/1
  saveData4/2 -> Mux/5
  saveData5/1 -> saveData6/2
  saveData/2 -> Mux/1
  saveData8/2 -> Mux/9
  data/1 -> saveData/2
  saveData7/2 -> Mux/8
  saveData/1 -> saveData1/2
  saveData9/2 -> Mux/10
  saveData6/1 -> saveData7/2
  saveData2/1 -> saveData3/2
  saveData5/2 -> Mux/6
  saveData1/1 -> saveData2/2
  saveData1/2 -> Mux/2
  saveBool/1 -> saveData/3, saveData1/3, saveData2/3, saveData3/3, saveData4/3, saveData5/3, saveData6/3, saveData7/3, saveData8/3, saveData9/3

== system D_20231120_Modell_Inbetriebnahme_BreakOutBox_Jetson/IO691/CAN Read Loop - Port 3/Enabled Subsystem/extract radar data from CAN msg stream/Subsystem1/Subsystem1 ==
  reset : Inport
  data : Inport  Port=2
  saveBool : Inport  Port=3
  Mux : Mux  Inputs=10
  saveData{,1..9} (10 alike) : lllalib/saveData  SystemSampleTime=-1  VariantActivationTime=update diagram  Latency=0  AutoFrameSizeCalculation=off
  out : Outport
  nextSave : Outport  Port=2
  wires:
  saveData3/2 -> Mux/4
  saveData8/1 -> saveData9/2
  saveData7/1 -> saveData8/2
  reset/1 -> saveData/1, saveData1/1, saveData2/1, saveData3/1, saveData4/1, saveData5/1, saveData6/1, saveData8/1, saveData9/1, saveData7/1
  saveData3/1 -> saveData4/2
  saveData4/1 -> saveData5/2
  saveData2/2 -> Mux/3
  Mux/1 -> out/1
  saveData6/2 -> Mux/7
  saveData9/1 -> nextSave/1
  saveData4/2 -> Mux/5
  saveData5/1 -> saveData6/2
  saveData/2 -> Mux/1
  saveData8/2 -> Mux/9
  data/1 -> saveData/2
  saveData7/2 -> Mux/8
  saveData/1 -> saveData1/2
  saveData9/2 -> Mux/10
  saveData6/1 -> saveData7/2
  saveData2/1 -> saveData3/2
  saveData5/2 -> Mux/6
  saveData1/1 -> saveData2/2
  saveData1/2 -> Mux/2
  saveBool/1 -> saveData/3, saveData1/3, saveData2/3, saveData3/3, saveData4/3, saveData5/3, saveData6/3, saveData7/3, saveData8/3, saveData9/3

== system D_20231120_Modell_Inbetriebnahme_BreakOutBox_Jetson/IO691/CAN Read Loop - Port 3/Enabled Subsystem/extract radar data from CAN msg stream/Subsystem1/Subsystem2 ==
  reset : Inport
  data : Inport  Port=2
  saveBool : Inport  Port=3
  Mux : Mux  Inputs=10
  saveData{,1..9} (10 alike) : lllalib/saveData  SystemSampleTime=-1  VariantActivationTime=update diagram  Latency=0  AutoFrameSizeCalculation=off
  out : Outport
  nextSave : Outport  Port=2
  wires:
  saveData3/2 -> Mux/4
  saveData8/1 -> saveData9/2
  saveData7/1 -> saveData8/2
  reset/1 -> saveData/1, saveData1/1, saveData2/1, saveData3/1, saveData4/1, saveData5/1, saveData6/1, saveData8/1, saveData9/1, saveData7/1
  saveData3/1 -> saveData4/2
  saveData4/1 -> saveData5/2
  saveData2/2 -> Mux/3
  Mux/1 -> out/1
  saveData6/2 -> Mux/7
  saveData9/1 -> nextSave/1
  saveData4/2 -> Mux/5
  saveData5/1 -> saveData6/2
  saveData/2 -> Mux/1
  saveData8/2 -> Mux/9
  data/1 -> saveData/2
  saveData7/2 -> Mux/8
  saveData/1 -> saveData1/2
  saveData9/2 -> Mux/10
  saveData6/1 -> saveData7/2
  saveData2/1 -> saveData3/2
  saveData5/2 -> Mux/6
  saveData1/1 -> saveData2/2
  saveData1/2 -> Mux/2
  saveBool/1 -> saveData/3, saveData1/3, saveData2/3, saveData3/3, saveData4/3, saveData5/3, saveData6/3, saveData7/3, saveData8/3, saveData9/3

== system D_20231120_Modell_Inbetriebnahme_BreakOutBox_Jetson/IO691/CAN Read Loop - Port 3/Enabled Subsystem/extract radar data from CAN msg stream/Subsystem1/Subsystem3 ==
  reset : Inport
  data : Inport  Port=2
  saveBool : Inport  Port=3
  Mux : Mux  Inputs=10
  saveData{,1..9} (10 alike) : lllalib/saveData  SystemSampleTime=-1  VariantActivationTime=update diagram  Latency=0  AutoFrameSizeCalculation=off
  out : Outport
  nextSave : Outport  Port=2
  wires:
  saveBool/1 -> saveData9/3, saveData8/3, saveData7/3, saveData6/3, saveData5/3, saveData4/3, saveData3/3, saveData2/3, saveData1/3, saveData/3
  saveData1/2 -> Mux/2
  saveData1/1 -> saveData2/2
  saveData5/2 -> Mux/6
  saveData2/1 -> saveData3/2
  saveData6/1 -> saveData7/2
  saveData9/2 -> Mux/10
  saveData/1 -> saveData1/2
  saveData7/2 -> Mux/8
  data/1 -> saveData/2
  saveData8/2 -> Mux/9
  saveData/2 -> Mux/1
  saveData5/1 -> saveData6/2
  saveData4/2 -> Mux/5
  saveData9/1 -> nextSave/1
  saveData6/2 -> Mux/7
  Mux/1 -> out/1
  saveData2/2 -> Mux/3
  saveData4/1 -> saveData5/2
  saveData3/1 -> saveData4/2
  reset/1 -> saveData7/1, saveData9/1, saveData8/1, saveData6/1, saveData5/1, saveData4/1, saveData3/1, saveData2/1, saveData1/1, saveData/1
  saveData7/1 -> saveData8/2
  saveData8/1 -> saveData9/2
  saveData3/2 -> Mux/4

== system D_20231120_Modell_Inbetriebnahme_BreakOutBox_Jetson/IO691/CAN Read Loop - Port 3/Enabled Subsystem/extract radar data from CAN msg stream/Subsystem1/Subsystem4 ==
  reset : Inport
  data : Inport  Port=2
  saveBool : Inport  Port=3
  Mux : Mux  Inputs=10
  saveData{,1..9} (10 alike) : lllalib/saveData  SystemSampleTime=-1  VariantActivationTime=update diagram  Latency=0  AutoFrameSizeCalculation=off
  out : Outport
  nextSave : Outport  Port=2
  wires:
  saveData3/2 -> Mux/4
  saveData8/1 -> saveData9/2
  saveData7/1 -> saveData8/2
  reset/1 -> saveData/1, saveData1/1, saveData2/1, saveData3/1, saveData4/1, saveData5/1, saveData6/1, saveData8/1, saveData9/1, saveData7/1
  saveData3/1 -> saveData4/2
  saveData4/1 -> saveData5/2
  saveData2/2 -> Mux/3
  Mux/1 -> out/1
  saveData6/2 -> Mux/7
  saveData9/1 -> nextSave/1
  saveData4/2 -> Mux/5
  saveData5/1 -> saveData6/2
  saveData/2 -> Mux/1
  saveData8/2 -> Mux/9
  data/1 -> saveData/2
  saveData7/2 -> Mux/8
  saveData/1 -> saveData1/2
  saveData9/2 -> Mux/10
  saveData6/1 -> saveData7/2
  saveData2/1 -> saveData3/2
  saveData5/2 -> Mux/6
  saveData1/1 -> saveData2/2
  saveData1/2 -> Mux/2
  saveBool/1 -> saveData/3, saveData1/3, saveData2/3, saveData3/3, saveData4/3, saveData5/3, saveData6/3, saveData7/3, saveData8/3, saveData9/3

== system D_20231120_Modell_Inbetriebnahme_BreakOutBox_Jetson/IO691/CAN Read Loop - Port 3/Enabled Subsystem/extract radar data from CAN msg stream/Subsystem1/Subsystem5 ==
  reset : Inport
  data : Inport  Port=2
  saveBool : Inport  Port=3
  Mux : Mux  Inputs=10
  saveData{,1..9} (10 alike) : lllalib/saveData  SystemSampleTime=-1  VariantActivationTime=update diagram  Latency=0  AutoFrameSizeCalculation=off
  out : Outport
  nextSave : Outport  Port=2
  wires:
  saveBool/1 -> saveData9/3, saveData8/3, saveData7/3, saveData6/3, saveData5/3, saveData4/3, saveData3/3, saveData2/3, saveData1/3, saveData/3
  saveData1/2 -> Mux/2
  saveData1/1 -> saveData2/2
  saveData5/2 -> Mux/6
  saveData2/1 -> saveData3/2
  saveData6/1 -> saveData7/2
  saveData9/2 -> Mux/10
  saveData/1 -> saveData1/2
  saveData7/2 -> Mux/8
  data/1 -> saveData/2
  saveData8/2 -> Mux/9
  saveData/2 -> Mux/1
  saveData5/1 -> saveData6/2
  saveData4/2 -> Mux/5
  saveData9/1 -> nextSave/1
  saveData6/2 -> Mux/7
  Mux/1 -> out/1
  saveData2/2 -> Mux/3
  saveData4/1 -> saveData5/2
  saveData3/1 -> saveData4/2
  reset/1 -> saveData7/1, saveData9/1, saveData8/1, saveData6/1, saveData5/1, saveData4/1, saveData3/1, saveData2/1, saveData1/1, saveData/1
  saveData7/1 -> saveData8/2
  saveData8/1 -> saveData9/2
  saveData3/2 -> Mux/4

== system D_20231120_Modell_Inbetriebnahme_BreakOutBox_Jetson/IO691/CAN Read Loop - Port 3/Enabled Subsystem/extract radar data from CAN msg stream/Subsystem1/Subsystem6 ==
  reset : Inport
  data : Inport  Port=2
  saveBool : Inport  Port=3
  Mux : Mux  Inputs=10
  saveData{,1..9} (10 alike) : lllalib/saveData  SystemSampleTime=-1  VariantActivationTime=update diagram  Latency=0  AutoFrameSizeCalculation=off
  out : Outport
  nextSave : Outport  Port=2
  wires:
  saveBool/1 -> saveData9/3, saveData8/3, saveData7/3, saveData6/3, saveData5/3, saveData4/3, saveData3/3, saveData2/3, saveData1/3, saveData/3
  saveData1/2 -> Mux/2
  saveData1/1 -> saveData2/2
  saveData5/2 -> Mux/6
  saveData2/1 -> saveData3/2
  saveData6/1 -> saveData7/2
  saveData9/2 -> Mux/10
  saveData/1 -> saveData1/2
  saveData7/2 -> Mux/8
  data/1 -> saveData/2
  saveData8/2 -> Mux/9
  saveData/2 -> Mux/1
  saveData5/1 -> saveData6/2
  saveData4/2 -> Mux/5
  saveData9/1 -> nextSave/1
  saveData6/2 -> Mux/7
  Mux/1 -> out/1
  saveData2/2 -> Mux/3
  saveData4/1 -> saveData5/2
  saveData3/1 -> saveData4/2
  reset/1 -> saveData7/1, saveData9/1, saveData8/1, saveData6/1, saveData5/1, saveData4/1, saveData3/1, saveData2/1, saveData1/1, saveData/1
  saveData7/1 -> saveData8/2
  saveData8/1 -> saveData9/2
  saveData3/2 -> Mux/4

== system D_20231120_Modell_Inbetriebnahme_BreakOutBox_Jetson/IO691/CAN Read Loop - Port 3/Enabled Subsystem/extract radar data from CAN msg stream/Subsystem1/Subsystem7 ==
  reset : Inport
  data : Inport  Port=2
  saveBool : Inport  Port=3
  Mux : Mux  Inputs=10
  saveData{,1..9} (10 alike) : lllalib/saveData  SystemSampleTime=-1  VariantActivationTime=update diagram  Latency=0  AutoFrameSizeCalculation=off
  out : Outport
  nextSave : Outport  Port=2
  wires:
  saveData3/2 -> Mux/4
  saveData8/1 -> saveData9/2
  saveData7/1 -> saveData8/2
  reset/1 -> saveData/1, saveData1/1, saveData2/1, saveData3/1, saveData4/1, saveData5/1, saveData6/1, saveData8/1, saveData9/1, saveData7/1
  saveData3/1 -> saveData4/2
  saveData4/1 -> saveData5/2
  saveData2/2 -> Mux/3
  Mux/1 -> out/1
  saveData6/2 -> Mux/7
  saveData9/1 -> nextSave/1
  saveData4/2 -> Mux/5
  saveData5/1 -> saveData6/2
  saveData/2 -> Mux/1
  saveData8/2 -> Mux/9
  data/1 -> saveData/2
  saveData7/2 -> Mux/8
  saveData/1 -> saveData1/2
  saveData9/2 -> Mux/10
  saveData6/1 -> saveData7/2
  saveData2/1 -> saveData3/2
  saveData5/2 -> Mux/6
  saveData1/1 -> saveData2/2
  saveData1/2 -> Mux/2
  saveBool/1 -> saveData/3, saveData1/3, saveData2/3, saveData3/3, saveData4/3, saveData5/3, saveData6/3, saveData7/3, saveData8/3, saveData9/3

== system D_20231120_Modell_Inbetriebnahme_BreakOutBox_Jetson/IO691/CAN Read Loop - Port 3/Enabled Subsystem/extract radar data from CAN msg stream/Subsystem1/Subsystem8 ==
  reset : Inport
  data : Inport  Port=2
  saveBool : Inport  Port=3
  Mux : Mux  Inputs=10
  saveData{,1..9} (10 alike) : lllalib/saveData  SystemSampleTime=-1  VariantActivationTime=update diagram  Latency=0  AutoFrameSizeCalculation=off
  out : Outport
  nextSave : Outport  Port=2
  wires:
  saveBool/1 -> saveData9/3, saveData8/3, saveData7/3, saveData6/3, saveData5/3, saveData4/3, saveData3/3, saveData2/3, saveData1/3, saveData/3
  saveData1/2 -> Mux/2
  saveData1/1 -> saveData2/2
  saveData5/2 -> Mux/6
  saveData2/1 -> saveData3/2
  saveData6/1 -> saveData7/2
  saveData9/2 -> Mux/10
  saveData/1 -> saveData1/2
  saveData7/2 -> Mux/8
  data/1 -> saveData/2
  saveData8/2 -> Mux/9
  saveData/2 -> Mux/1
  saveData5/1 -> saveData6/2
  saveData4/2 -> Mux/5
  saveData9/1 -> nextSave/1
  saveData6/2 -> Mux/7
  Mux/1 -> out/1
  saveData2/2 -> Mux/3
  saveData4/1 -> saveData5/2
  saveData3/1 -> saveData4/2
  reset/1 -> saveData7/1, saveData9/1, saveData8/1, saveData6/1, saveData5/1, saveData4/1, saveData3/1, saveData2/1, saveData1/1, saveData/1
  saveData7/1 -> saveData8/2
  saveData8/1 -> saveData9/2
  saveData3/2 -> Mux/4

== system D_20231120_Modell_Inbetriebnahme_BreakOutBox_Jetson/IO691/CAN Read Loop - Port 3/Enabled Subsystem/extract radar data from CAN msg stream/Subsystem1/Subsystem9 ==
  reset : Inport
  data : Inport  Port=2
  saveBool : Inport  Port=3
  Mux : Mux  Inputs=10
  saveData{,1..9} (10 alike) : lllalib/saveData  SystemSampleTime=-1  VariantActivationTime=update diagram  Latency=0  AutoFrameSizeCalculation=off
  out : Outport
  nextSave : Outport  Port=2
  wires:
  saveData3/2 -> Mux/4
  saveData8/1 -> saveData9/2
  saveData7/1 -> saveData8/2
  reset/1 -> saveData/1, saveData1/1, saveData2/1, saveData3/1, saveData4/1, saveData5/1, saveData6/1, saveData8/1, saveData9/1, saveData7/1
  saveData3/1 -> saveData4/2
  saveData4/1 -> saveData5/2
  saveData2/2 -> Mux/3
  Mux/1 -> out/1
  saveData6/2 -> Mux/7
  saveData9/1 -> nextSave/1
  saveData4/2 -> Mux/5
  saveData5/1 -> saveData6/2
  saveData/2 -> Mux/1
  saveData8/2 -> Mux/9
  data/1 -> saveData/2
  saveData7/2 -> Mux/8
  saveData/1 -> saveData1/2
  saveData9/2 -> Mux/10
  saveData6/1 -> saveData7/2
  saveData2/1 -> saveData3/2
  saveData5/2 -> Mux/6
  saveData1/1 -> saveData2/2
  saveData1/2 -> Mux/2
  saveBool/1 -> saveData/3, saveData1/3, saveData2/3, saveData3/3, saveData4/3, saveData5/3, saveData6/3, saveData7/3, saveData8/3, saveData9/3

== system D_20231120_Modell_Inbetriebnahme_BreakOutBox_Jetson/IO691/CAN Read Loop - Port 3/Enabled Subsystem/extract radar data from CAN msg stream/Subsystem100/Subsystem ==
  reset : Inport
  data : Inport  Port=2
  saveBool : Inport  Port=3
  Mux : Mux  Inputs=10
  saveData{,1..9} (10 alike) : lllalib/saveData  SystemSampleTime=-1  VariantActivationTime=update diagram  Latency=0  AutoFrameSizeCalculation=off
  out : Outport
  nextSave : Outport  Port=2
  wires:
  saveData3/2 -> Mux/4
  saveData8/1 -> saveData9/2
  saveData7/1 -> saveData8/2
  reset/1 -> saveData/1, saveData1/1, saveData2/1, saveData3/1, saveData4/1, saveData5/1, saveData6/1, saveData8/1, saveData9/1, saveData7/1
  saveData3/1 -> saveData4/2
  saveData4/1 -> saveData5/2
  saveData2/2 -> Mux/3
  Mux/1 -> out/1
  saveData6/2 -> Mux/7
  saveData9/1 -> nextSave/1
  saveData4/2 -> Mux/5
  saveData5/1 -> saveData6/2
  saveData/2 -> Mux/1
  saveData8/2 -> Mux/9
  data/1 -> saveData/2
  saveData7/2 -> Mux/8
  saveData/1 -> saveData1/2
  saveData9/2 -> Mux/10
  saveData6/1 -> saveData7/2
  saveData2/1 -> saveData3/2
  saveData5/2 -> Mux/6
  saveData1/1 -> saveData2/2
  saveData1/2 -> Mux/2
  saveBool/1 -> saveData/3, saveData1/3, saveData2/3, saveData3/3, saveData4/3, saveData5/3, saveData6/3, saveData7/3, saveData8/3, saveData9/3

== system D_20231120_Modell_Inbetriebnahme_BreakOutBox_Jetson/IO691/CAN Read Loop - Port 3/Enabled Subsystem/extract radar data from CAN msg stream/Subsystem100/Subsystem1 ==
  reset : Inport
  data : Inport  Port=2
  saveBool : Inport  Port=3
  Mux : Mux  Inputs=10
  saveData{,1..9} (10 alike) : lllalib/saveData  SystemSampleTime=-1  VariantActivationTime=update diagram  Latency=0  AutoFrameSizeCalculation=off
  out : Outport
  nextSave : Outport  Port=2
  wires:
  saveData3/2 -> Mux/4
  saveData8/1 -> saveData9/2
  saveData7/1 -> saveData8/2
  reset/1 -> saveData/1, saveData1/1, saveData2/1, saveData3/1, saveData4/1, saveData5/1, saveData6/1, saveData8/1, saveData9/1, saveData7/1
  saveData3/1 -> saveData4/2
  saveData4/1 -> saveData5/2
  saveData2/2 -> Mux/3
  Mux/1 -> out/1
  saveData6/2 -> Mux/7
  saveData9/1 -> nextSave/1
  saveData4/2 -> Mux/5
  saveData5/1 -> saveData6/2
  saveData/2 -> Mux/1
  saveData8/2 -> Mux/9
  data/1 -> saveData/2
  saveData7/2 -> Mux/8
  saveData/1 -> saveData1/2
  saveData9/2 -> Mux/10
  saveData6/1 -> saveData7/2
  saveData2/1 -> saveData3/2
  saveData5/2 -> Mux/6
  saveData1/1 -> saveData2/2
  saveData1/2 -> Mux/2
  saveBool/1 -> saveData/3, saveData1/3, saveData2/3, saveData3/3, saveData4/3, saveData5/3, saveData6/3, saveData7/3, saveData8/3, saveData9/3

== system D_20231120_Modell_Inbetriebnahme_BreakOutBox_Jetson/IO691/CAN Read Loop - Port 3/Enabled Subsystem/extract radar data from CAN msg stream/Subsystem100/Subsystem2 ==
  reset : Inport
  data : Inport  Port=2
  saveBool : Inport  Port=3
  Mux : Mux  Inputs=10
  saveData{,1..9} (10 alike) : lllalib/saveData  SystemSampleTime=-1  VariantActivationTime=update diagram  Latency=0  AutoFrameSizeCalculation=off
  out : Outport
  nextSave : Outport  Port=2
  wires:
  saveData3/2 -> Mux/4
  saveData8/1 -> saveData9/2
  saveData7/1 -> saveData8/2
  reset/1 -> saveData/1, saveData1/1, saveData2/1, saveData3/1, saveData4/1, saveData5/1, saveData6/1, saveData8/1, saveData9/1, saveData7/1
  saveData3/1 -> saveData4/2
  saveData4/1 -> saveData5/2
  saveData2/2 -> Mux/3
  Mux/1 -> out/1
  saveData6/2 -> Mux/7
  saveData9/1 -> nextSave/1
  saveData4/2 -> Mux/5
  saveData5/1 -> saveData6/2
  saveData/2 -> Mux/1
  saveData8/2 -> Mux/9
  data/1 -> saveData/2
  saveData7/2 -> Mux/8
  saveData/1 -> saveData1/2
  saveData9/2 -> Mux/10
  saveData6/1 -> saveData7/2
  saveData2/1 -> saveData3/2
  saveData5/2 -> Mux/6
  saveData1/1 -> saveData2/2
  saveData1/2 -> Mux/2
  saveBool/1 -> saveData/3, saveData1/3, saveData2/3, saveData3/3, saveData4/3, saveData5/3, saveData6/3, saveData7/3, saveData8/3, saveData9/3

== system D_20231120_Modell_Inbetriebnahme_BreakOutBox_Jetson/IO691/CAN Read Loop - Port 3/Enabled Subsystem/extract radar data from CAN msg stream/Subsystem100/Subsystem3 ==
  reset : Inport
  data : Inport  Port=2
  saveBool : Inport  Port=3
  Mux : Mux  Inputs=10
  saveData{,1..9} (10 alike) : lllalib/saveData  SystemSampleTime=-1  VariantActivationTime=update diagram  Latency=0  AutoFrameSizeCalculation=off
  out : Outport
  nextSave : Outport  Port=2
  wires:
  saveBool/1 -> saveData9/3, saveData8/3, saveData7/3, saveData6/3, saveData5/3, saveData4/3, saveData3/3, saveData2/3, saveData1/3, saveData/3
  saveData1/2 -> Mux/2
  saveData1/1 -> saveData2/2
  saveData5/2 -> Mux/6
  saveData2/1 -> saveData3/2
  saveData6/1 -> saveData7/2
  saveData9/2 -> Mux/10
  saveData/1 -> saveData1/2
  saveData7/2 -> Mux/8
  data/1 -> saveData/2
  saveData8/2 -> Mux/9
  saveData/2 -> Mux/1
  saveData5/1 -> saveData6/2
  saveData4/2 -> Mux/5
  saveData9/1 -> nextSave/1
  saveData6/2 -> Mux/7
  Mux/1 -> out/1
  saveData2/2 -> Mux/3
  saveData4/1 -> saveData5/2
  saveData3/1 -> saveData4/2
  reset/1 -> saveData7/1, saveData9/1, saveData8/1, saveData6/1, saveData5/1, saveData4/1, saveData3/1, saveData2/1, saveData1/1, saveData/1
  saveData7/1 -> saveData8/2
  saveData8/1 -> saveData9/2
  saveData3/2 -> Mux/4
